simulink model "trackVehicleNewVer7_SonarPath"  (R2018b)
settings: Solver=ode45  StartTime=0.0  StopTime=100  FixedStep=0.1  RelTol=1e-3  EnableMultiTasking=on
PreLoadFcn:
  | RTWConfigurationCB('preloadfcn', bdroot);
InitFcn:
  | parameterVehicle
  | parameterObstacles
  | parameterGNC
  | parameterOccupancyGrid
  | parameterPathPlanner
  | parameterWaypointGenerator
  | miscParameters
StopFcn:
  | myAnimationSonarPath(xActEst,yActEst,thetaActEst,X_array, Y_array, rp1,rp2,sonarInfo, obstaclesArray, OccGrid, gridorig, cellsize)
values from neighbouring files (symbols this model uses):
  b = 0.32    [parameterVehicle.m]
  bDR = b    [parameterGNC.m]
  dcArray = [-uv -un-1 -un 0 un un+1 uv]    [parameterVehicle.m]
  dcArrayDR = [-uv -un-1 -un 0 un un+1 uv]    [parameterGNC.m]
  eTick = 1050    [parameterVehicle.m]
  eTickDR = eTick    [parameterGNC.m]
  KP1 = 8    [parameterGNC.m]
  KP2 = 20    [parameterGNC.m]
  maxgoaldist = 0.3    [parameterWaypointGenerator.m]
  maxwaydist = 0.5    [parameterWaypointGenerator.m]
  rl = 1*rNominal    (= 0.06)    [parameterVehicle.m]
  rNominal = 0.06    [parameterVehicle.m]
  rNominalDR = rNominal    [parameterGNC.m]
  rp1 = 0.3    [parameterGNC.m]
  rr = 1*rNominal    (= 0.06)    [parameterVehicle.m]
  Tau1 = 0.01    [parameterGNC.m]
  Tau2 = 0.1    [parameterGNC.m]
  TauEncoderDR = 0.1    [parameterGNC.m]
  thetaIC = 0*(pi/180)    (= 0)    [parameterVehicle.m]
  Tsample = 1/10    (= 0.1)    [parameterGNC.m]
  TsampleEncoder = 1/10    (= 0.1)    [parameterVehicle.m]
  TsampleEncoderDR = TsampleEncoder    [parameterGNC.m]
  Vcom = 1.5    [parameterGNC.m]
  wArray = [-Vmax, -Vmin, 0, 0,   0, Vmin, Vmax]./rNominal    [parameterVehicle.m]
  wArrayDR = [-Vmax, -Vmin, -Vmin/100, 0,   Vmin/100, Vmin, Vmax]./rNominal    [parameterGNC.m]
  xIC = 0    [parameterVehicle.m]
  yIC = 0    [parameterVehicle.m]
undefined symbols (not defined in the file or in its folder): DiscIntNeverNeededParam, obstaclesArray, sonar, X, Y, Z
libraries: robotlib x24, simulink x10, aerolibanimutils x1
CloseFcn:
  | rtwprivate ssgencode ModelCloseRequest track_vehicle6_v2
settings Model: Creator=Dogan  LastModifiedBy=uvs2
settings DataIOCC: LimitDataPoints=on  SaveFormat=Array  SignalLoggingSaveFormat=ModelDataLogs
settings OptimizationCC: ExpressionDepthLimit=2147483647  InitFltsAndDblsToZero=on  LifeSpan=inf
settings DebuggingCC: SaveWithParameterizedLinksMsg=none  UnderspecifiedInitializationDetection=Classic  MergeDetectMultiDrivingBlocksExec=none  SignalResolutionControl=TryResolveAllWithWarning  SolverPrmCheckMsg=warning  MultiTaskDSMMsg=warning  MultiTaskCondExecSysMsg=none  FcnCallInpInsideContextMsg=warning  StateNameClashWarn=warning  SFUnexpectedBacktrackingDiag=warning  SFNoUnconditionalDefaultTransitionDiag=warning  SFExecutionAtInitializationDiag=none
settings HardwareCC: ProdBitPerLong=64  ProdLargestAtomicFloat=None  ProdHWDeviceType=Intel->x86-64  TargetHWDeviceType=32-bit Generic
settings ModelReferenceCC: PropagateSignalLabelsOutOfModel=off
settings SFSimCC: SimUseLocalCustomCode=off  SimParseCustomCode=off
settings RTWCC: Description=Generic Real-Time Target  RTWUseLocalCustomCode=off
settings CodeAppCC: GenerateComments=off  SimulinkBlockComments=off
settings GRTTargetCC: TargetLangStandard=C89/C90 (ANSI)  GeneratePreprocessorConditionals=Disable all
settings ConfigComp: CovMetricSettings=dw  CovHtmlReporting=on  CovSaveCumulativeToWorkspaceVar=on  CovSaveSingleToWorkspaceVar=on  CovExternalEMLEnable=off

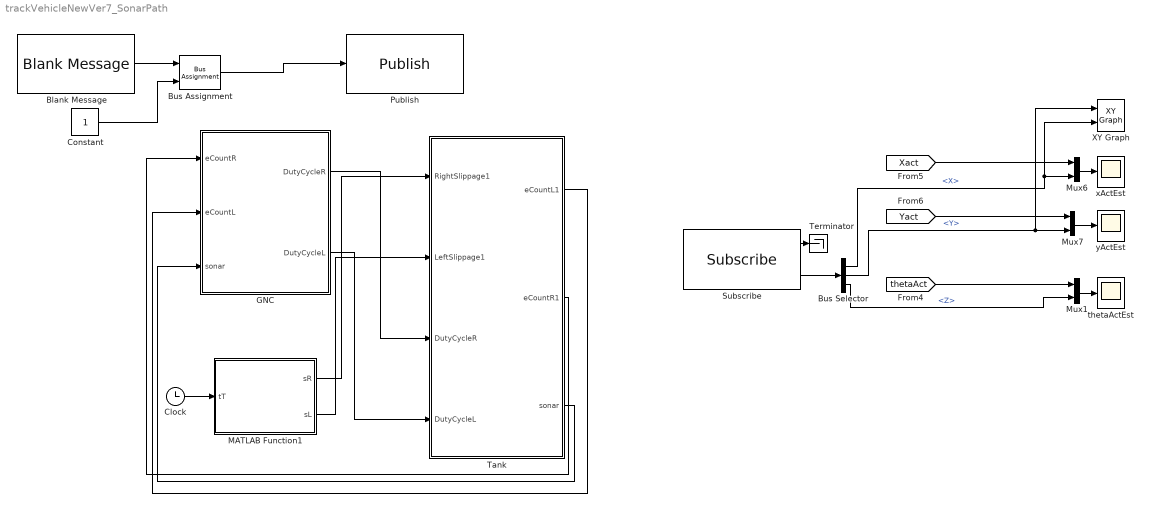
== system trackVehicleNewVer7_SonarPath ==
  Blank Message : robotlib/Blank Message  messageClass=Message  entityType=std_msgs/Bool  messageType=std_msgs/Bool  SampleTime=-1
      settings: SourceProductBaseCode=RO
  Bus Assignment : BusAssignment  AssignedSignals=Data
  Bus Selector : BusSelector  OutputSignals=X,Y,Z
  Clock : Clock
  Constant : Constant  OutDataTypeStr=boolean
  GNC : Subsystem
  MATLAB Function1 : MATLAB Function  TreatAsAtomicUnit=on
  Mux1 : Mux  Inputs=2
  Mux6 : Mux  Inputs=2
  Mux7 : Mux  Inputs=2
  Publish : robotlib/Publish  topicSource=Specify your own  topic=/start  messageType=std_msgs/Bool  messageQueueLength=1
      settings: SourceProductBaseCode=RO
  Subscribe : robotlib/Subscribe  topicSource=Specify your own  topic=/odometry  messageType=geometry_msgs/Point  sampleTime=-1  messageQueueLength=1
      settings: SourceProductBaseCode=RO
  Tank : Subsystem
  Terminator : Terminator
  XY Graph : simulink/Sinks/XY Graph  xmin=-1  xmax=9  ymin=-1  ymax=9  st=-1
  thetaActEst : Scope
  xActEst : Scope
  yActEst : Scope
  wires:
  Clock/1 -> MATLAB Function1/1(tT)
  Bus Selector/1 -> XY Graph/2, Mux6/2  "<X>"
  Mux6/1 -> xActEst/1
  Bus Selector/2 -> Mux7/2, XY Graph/1  "<Y>"
  [Xact] -> Mux6/1
  [Yact] -> Mux7/1
  Mux7/1 -> yActEst/1
  Bus Selector/3 -> Mux1/2  "<Z>"
  Mux1/1 -> thetaActEst/1
  [thetaAct] -> Mux1/1
  Subscribe/2 -> Bus Selector/1
  Blank Message/1 -> Bus Assignment/1
  Bus Assignment/1 -> Publish/1
  Constant/1 -> Bus Assignment/2
  Subscribe/1 -> Terminator/1
  GNC/1(DutyCycleR) -> Tank/3(DutyCycleR)
  GNC/2(DutyCycleL) -> Tank/4(DutyCycleL)
  MATLAB Function1/1(sR) -> Tank/1(RightSlippage1)
  MATLAB Function1/2(sL) -> Tank/2(LeftSlippage1)
  Tank/3(sonar) -> GNC/3(sonar)
  Tank/2("eCountR1 ") -> GNC/1(eCountR)
  Tank/1(eCountL1) -> GNC/2(eCountL)

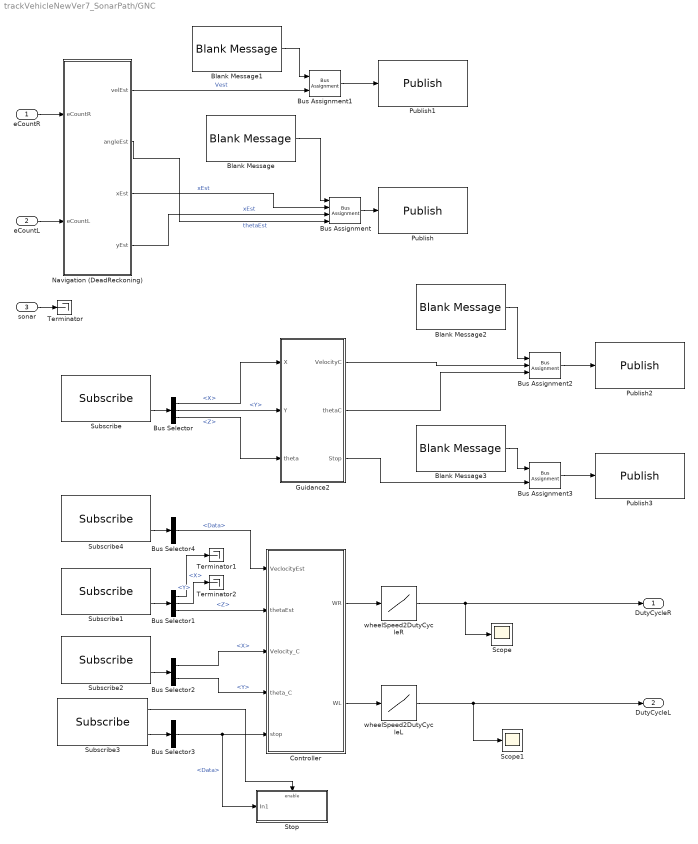
== system trackVehicleNewVer7_SonarPath/GNC ==
  eCountR : Inport
  eCountL : Inport  Port=2
  sonar : Inport  Port=3
  Blank Message : robotlib/Blank Message  messageClass=Message  entityType=geometry_msgs/Point  messageType=geometry_msgs/Point  SampleTime=inf
      settings: SourceProductBaseCode=RO
  Blank Message1 : robotlib/Blank Message  messageClass=Message  entityType=std_msgs/Float64  messageType=std_msgs/Float64  SampleTime=inf
      settings: SourceProductBaseCode=RO
  Blank Message2 : robotlib/Blank Message  messageClass=Message  entityType=geometry_msgs/Point  messageType=geometry_msgs/Point  SampleTime=inf
      settings: SourceProductBaseCode=RO
  Blank Message3 : robotlib/Blank Message  messageClass=Message  entityType=std_msgs/Bool  messageType=std_msgs/Bool  SampleTime=inf
      settings: SourceProductBaseCode=RO
  Bus Assignment : BusAssignment  AssignedSignals=X,Y,Z
  Bus Assignment1 : BusAssignment  AssignedSignals=Data
  Bus Assignment2 : BusAssignment  AssignedSignals=X,Y
  Bus Assignment3 : BusAssignment  AssignedSignals=Data
  Bus Selector : BusSelector  OutputSignals=X,Y,Z
  Bus Selector1 : BusSelector  OutputSignals=X,Y,Z
  Bus Selector2 : BusSelector  OutputSignals=X,Y
  Bus Selector3 : BusSelector  OutputSignals=Data
  Bus Selector4 : BusSelector  OutputSignals=Data
  Controller : Subsystem
  Guidance2 : Subsystem
  Navigation (DeadReckoning) : Subsystem
  Publish : robotlib/Publish  topicSource=Specify your own  topic=/odometry  messageType=geometry_msgs/Point  messageQueueLength=1
      settings: SourceProductBaseCode=RO
  Publish1 : robotlib/Publish  topicSource=Specify your own  topic=/velEst  messageType=std_msgs/Float64  messageQueueLength=1
      settings: SourceProductBaseCode=RO
  Publish2 : robotlib/Publish  topicSource=Specify your own  topic=/controlcommands  messageType=geometry_msgs/Point  messageQueueLength=1
      settings: SourceProductBaseCode=RO
  Publish3 : robotlib/Publish  topicSource=Specify your own  topic=/stop  messageType=std_msgs/Bool  messageQueueLength=1
      settings: SourceProductBaseCode=RO
  Scope : Scope
  Scope1 : Scope
  Stop : Subsystem  TreatAsAtomicUnit=on
  Subscribe : robotlib/Subscribe  topicSource=Specify your own  topic=/odometry  messageType=geometry_msgs/Point  sampleTime=-1  messageQueueLength=1
      settings: SourceProductBaseCode=RO
  Subscribe1 : robotlib/Subscribe  topicSource=Specify your own  topic=/odometry  messageType=geometry_msgs/Point  sampleTime=-1  messageQueueLength=1
      settings: SourceProductBaseCode=RO
  Subscribe2 : robotlib/Subscribe  topicSource=Specify your own  topic=/controlcommands  messageType=geometry_msgs/Point  sampleTime=-1  messageQueueLength=1
      settings: SourceProductBaseCode=RO
  Subscribe3 : robotlib/Subscribe  topicSource=Specify your own  topic=/stop  messageType=std_msgs/Bool  sampleTime=-1  messageQueueLength=1
      settings: SourceProductBaseCode=RO
  Subscribe4 : robotlib/Subscribe  topicSource=Specify your own  topic=/velEst  messageType=std_msgs/Float64  sampleTime=-1  messageQueueLength=1
      settings: SourceProductBaseCode=RO
  Terminator : Terminator
  Terminator1 : Terminator
  Terminator2 : Terminator
  wheelSpeed2DutyCycleL : Lookup  InputValues=wArrayDR  Table=dcArrayDR  LookUpMeth=Interpolation-Use End Values
  wheelSpeed2DutyCycleR : Lookup  InputValues=wArrayDR  Table=dcArrayDR  LookUpMeth=Interpolation-Use End Values
  DutyCycleR : Outport
  DutyCycleL : Outport  Port=2
  wires:
  Controller/2(WL) -> wheelSpeed2DutyCycleL/1
  Guidance2/2(thetaC) -> Bus Assignment2/3
  Guidance2/1(VelocityC) -> Bus Assignment2/2
  eCountR/1 -> Navigation (DeadReckoning)/1(eCountR)
  eCountL/1 -> Navigation (DeadReckoning)/2(eCountL)
  Navigation (DeadReckoning)/1(velEst) -> Bus Assignment1/2  "Vest"
  Navigation (DeadReckoning)/2(angleEst) -> Bus Assignment/4  "thetaEst"
  Navigation (DeadReckoning)/3(xEst) -> Bus Assignment/2  "xEst"
  Navigation (DeadReckoning)/4(yEst) -> Bus Assignment/3  "xEst"
  Controller/1(WR) -> wheelSpeed2DutyCycleR/1
  Guidance2/3(Stop) -> Bus Assignment3/2
  sonar/1 -> Terminator/1
  Bus Assignment/1 -> Publish/1
  Blank Message/1 -> Bus Assignment/1
  Blank Message1/1 -> Bus Assignment1/1
  Bus Assignment1/1 -> Publish1/1
  Subscribe/2 -> Bus Selector/1
  Bus Selector/1 -> Guidance2/1(X)  "<X>"
  Bus Selector/2 -> Guidance2/2(Y)  "<Y>"
  Bus Selector/3 -> Guidance2/3(theta)  "<Z>"
  Bus Assignment2/1 -> Publish2/1
  Blank Message2/1 -> Bus Assignment2/1
  Subscribe1/2 -> Bus Selector1/1
  Bus Selector1/3 -> Controller/2(thetaEst)  "<Z>"
  Bus Selector1/1 -> Terminator1/1  "<X>"
  Bus Selector1/2 -> Terminator2/1  "<Y>"
  Subscribe2/2 -> Bus Selector2/1
  Bus Selector2/1 -> Controller/3(Velocity_C)  "<X>"
  Bus Selector2/2 -> Controller/4(theta_C)  "<Y>"
  Bus Assignment3/1 -> Publish3/1
  Blank Message3/1 -> Bus Assignment3/1
  Subscribe3/2 -> Bus Selector3/1
  Bus Selector3/1 -> Stop/1(In1), Controller/5(stop)  "<Data>"
  Subscribe4/2 -> Bus Selector4/1
  Bus Selector4/1 -> Controller/1(VeclocityEst)  "<Data>"
  Subscribe3/1 -> Stop/Enable
  wheelSpeed2DutyCycleR/1 -> Scope/1, DutyCycleR/1
  wheelSpeed2DutyCycleL/1 -> Scope1/1, DutyCycleL/1

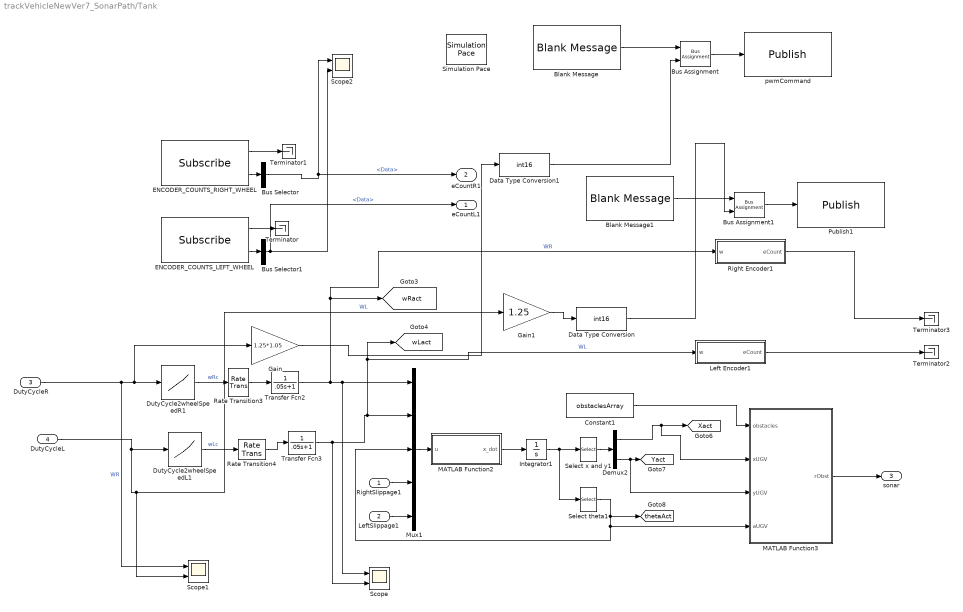
== system trackVehicleNewVer7_SonarPath/Tank ==
  RightSlippage1 : Inport
  LeftSlippage1 : Inport  Port=2
  DutyCycleR : Inport  Port=3
  DutyCycleL : Inport  Port=4
  Blank Message : robotlib/Blank Message  messageClass=Message  entityType=std_msgs/Int16  messageType=std_msgs/Int16  SampleTime=inf
      settings: SourceProductBaseCode=RO
  Blank Message1 : robotlib/Blank Message  messageClass=Message  entityType=std_msgs/Int16  messageType=std_msgs/Int16  SampleTime=inf
      settings: SourceProductBaseCode=RO
  Bus Assignment : BusAssignment  AssignedSignals=Data
  Bus Assignment1 : BusAssignment  AssignedSignals=Data
  Bus Selector : BusSelector  OutputSignals=Data
  Bus Selector1 : BusSelector  OutputSignals=Data
  Constant1 : Constant  Value=obstaclesArray
  Data Type Conversion : DataTypeConversion  OutDataTypeStr=int16
  Data Type Conversion1 : DataTypeConversion  OutDataTypeStr=int16
  Demux2 : Demux  Outputs=2
  DutyCycle2wheelSpeedL1 : Lookup  InputValues=dcArray  Table=wArray  LookUpMeth=Interpolation-Use End Values
  DutyCycle2wheelSpeedR1 : Lookup  InputValues=dcArray  Table=wArray  LookUpMeth=Interpolation-Use End Values
  ENCODER_COUNTS_LEFT_WHEEL : robotlib/Subscribe  topicSource=Select from ROS network  topic=/enco_L  messageType=std_msgs/Int16  sampleTime=-1  messageQueueLength=1
      settings: SourceProductBaseCode=RO
  ENCODER_COUNTS_RIGHT_WHEEL : robotlib/Subscribe  topicSource=Select from ROS network  topic=/enco_R  messageType=std_msgs/Int16  sampleTime=-1  messageQueueLength=1
      settings: SourceProductBaseCode=RO
  Gain : Gain  Gain=1.25*1.05
  Gain1 : Gain  Gain=1.25
  Integrator1 : Integrator  InitialCondition=[xIC; yIC ; thetaIC]
  Left Encoder1 : Subsystem
  MATLAB Function2 : MATLAB Function  TreatAsAtomicUnit=on
  MATLAB Function3 : MATLAB Function  TreatAsAtomicUnit=on  SystemSampleTime=sonar.Ts
  Mux1 : Mux  Inputs=5
  Publish1 : robotlib/Publish  topicSource=Select from ROS network  topic=/pwm_cmd_l  messageType=std_msgs/Int16  messageQueueLength=1
      settings: SourceProductBaseCode=RO
  Rate Transition3 : RateTransition
  Rate Transition4 : RateTransition  OutPortSampleTimeOpt=Inherit
  Right Encoder1 : Subsystem
  Scope : Scope  NumInputPorts=2
  Scope1 : Scope  NumInputPorts=2
  Scope2 : Scope  NumInputPorts=2
  Select theta1 : Selector  InputPortWidth=3  IndexOptions=Index vector (dialog)  Indices=3  OutputSizes=1
  Select x and y1 : Selector  InputPortWidth=3  IndexOptions=Index vector (dialog)  Indices=[1 2]  OutputSizes=1
  Simulation Pace : aerolibanimutils/Simulation Pace  SimulationPace=1  SleepMode=MATLAB Thread  OutputPaceError=off  SampleTime=1/30
  Terminator{,1..3} (4 alike) : Terminator
  Transfer Fcn2 : TransferFcn  Denominator=[.05 1]
  Transfer Fcn3 : TransferFcn  Denominator=[.05 1]
  pwmCommand : robotlib/Publish  topicSource=Select from ROS network  topic=/pwm_cmd_r  messageType=std_msgs/Int16  messageQueueLength=1
      settings: SourceProductBaseCode=RO
  eCountL1 : Outport
  "eCountR1 " : Outport  Port=2
  sonar : Outport  Port=3
  tag scope: Xact=global, Yact=global, thetaAct=global, wLact=global, wRact=global
  wires:
  Select theta1/1 -> MATLAB Function3/4(aUGV), Mux1/3, [thetaAct]
  Demux2/1 -> MATLAB Function3/2(xUGV), [Xact]
  Data Type Conversion1/1 -> Bus Assignment/2
  Data Type Conversion/1 -> Bus Assignment1/2
  DutyCycleL/1 -> DutyCycle2wheelSpeedL1/1, Scope1/2, Gain1/1  "WL"
  RightSlippage1/1 -> Mux1/4
  Left Encoder1/1(eCount) -> Terminator2/1
  Rate Transition4/1 -> Transfer Fcn3/1
  Mux1/1 -> MATLAB Function2/1(u)
  Gain1/1 -> Data Type Conversion/1
  Blank Message/1 -> Bus Assignment/1
  ENCODER_COUNTS_LEFT_WHEEL/2 -> Bus Selector1/1
  Demux2/2 -> MATLAB Function3/3(yUGV), [Yact]
  LeftSlippage1/1 -> Mux1/5
  DutyCycle2wheelSpeedL1/1 -> Rate Transition4/1  "wLc"
  Transfer Fcn3/1 -> Scope/2, Left Encoder1/1(w), [wLact], Mux1/2  "WL"
  ENCODER_COUNTS_RIGHT_WHEEL/2 -> Bus Selector/1
  Gain/1 -> Data Type Conversion1/1
  Bus Assignment1/1 -> Publish1/1
  Blank Message1/1 -> Bus Assignment1/1
  ENCODER_COUNTS_RIGHT_WHEEL/1 -> Terminator1/1
  Bus Assignment/1 -> pwmCommand/1
  Transfer Fcn2/1 -> [wRact], Right Encoder1/1(w), Scope/1, Mux1/1  "WR"
  Rate Transition3/1 -> Transfer Fcn2/1
  Integrator1/1 -> Select theta1/1, Select x and y1/1
  Bus Selector1/1 -> Scope2/2, eCountL1/1  "<Data>"
  MATLAB Function2/1(x_dot) -> Integrator1/1
  DutyCycleR/1 -> Scope1/1, Gain/1, DutyCycle2wheelSpeedR1/1  "WR"
  Bus Selector/1 -> "eCountR1 "/1, Scope2/1  "<Data>"
  ENCODER_COUNTS_LEFT_WHEEL/1 -> Terminator/1
  Right Encoder1/1(eCount) -> Terminator3/1
  DutyCycle2wheelSpeedR1/1 -> Rate Transition3/1  "wRc"
  Select x and y1/1 -> Demux2/1
  Constant1/1 -> MATLAB Function3/1(obstacles)
  MATLAB Function3/1(rObst) -> sonar/1

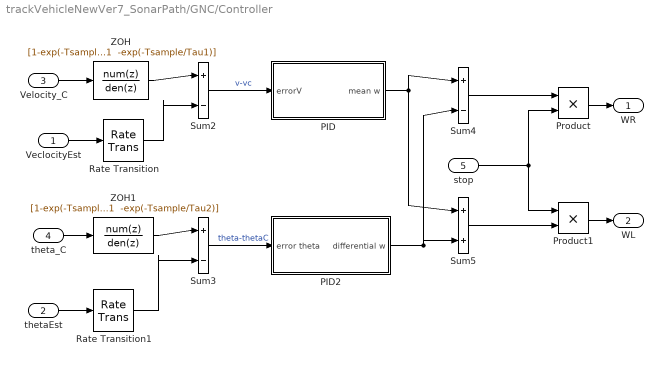
== system trackVehicleNewVer7_SonarPath/GNC/Controller ==
  VeclocityEst : Inport
  thetaEst : Inport  Port=2
  Velocity_C : Inport  Port=3
  theta_C : Inport  Port=4
  stop : Inport  Port=5
  PID : Subsystem
  PID2 : Subsystem
  Product : Product  RndMeth=Zero
  Product1 : Product  RndMeth=Zero
  Rate Transition : RateTransition  Deterministic=off
  Rate Transition1 : RateTransition  Deterministic=off
  Sum2 : Sum  Inputs=|+|-|  SampleTime=Tsample
  Sum3 : Sum  Inputs=|+|-|  SampleTime=Tsample
  Sum4 : Sum  Inputs=+|-
  Sum5 : Sum  Inputs=+|+
  ZOH : DiscreteTransferFcn  Numerator=[1-exp(-Tsample/Tau1)]  Denominator="[1  -exp(-Tsample/Tau1)]"  SampleTime=Tsample
  ZOH1 : DiscreteTransferFcn  Numerator=[1-exp(-Tsample/Tau2)]  Denominator="[1  -exp(-Tsample/Tau2)]"  SampleTime=Tsample
  WR : Outport
  WL : Outport  Port=2
  wires:
  Rate Transition1/1 -> Sum3/2
  ZOH1/1 -> Sum3/1
  Rate Transition/1 -> Sum2/2
  ZOH/1 -> Sum2/1
  Sum3/1 -> PID2/1(error theta)  "theta-thetaC"
  Sum2/1 -> PID/1(errorV)  "v-vc"
  VeclocityEst/1 -> Rate Transition/1
  Velocity_C/1 -> ZOH/1
  thetaEst/1 -> Rate Transition1/1
  theta_C/1 -> ZOH1/1
  PID/1(mean w) -> Sum4/1, Sum5/1
  PID2/1(differential w) -> Sum4/2, Sum5/2
  Sum4/1 -> Product/1
  stop/1 -> Product1/1, Product/2
  Sum5/1 -> Product1/2
  Product/1 -> WR/1
  Product1/1 -> WL/1

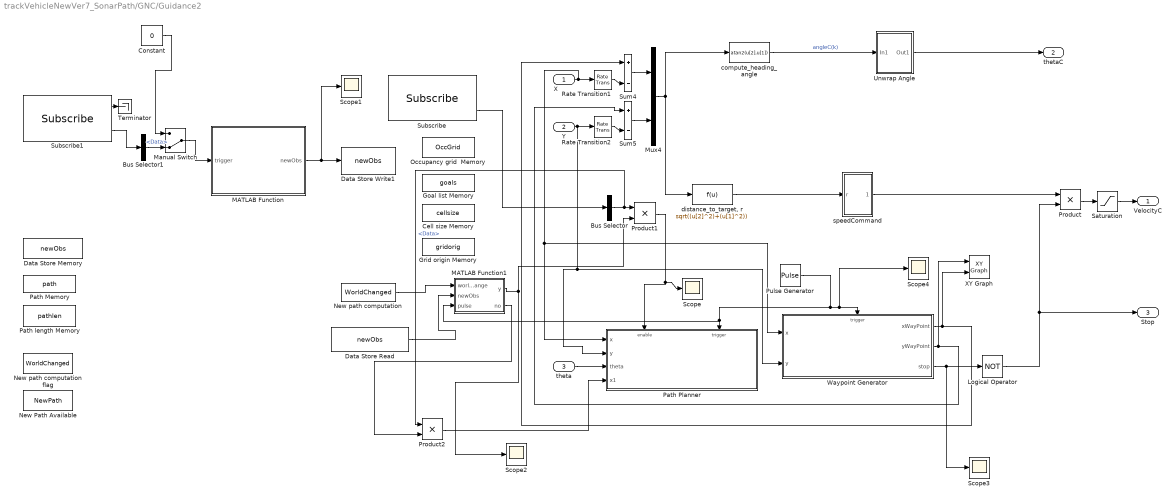
== system trackVehicleNewVer7_SonarPath/GNC/Guidance2 ==
  X : Inport
  Y : Inport  Port=2
  theta : Inport  Port=3
  Bus Selector : BusSelector  OutputSignals=Data
  Bus Selector1 : BusSelector  OutputSignals=Data
  Cell size Memory : DataStoreMemory  DataStoreName=cellsize  ReadBeforeWriteMsg=warning  WriteAfterWriteMsg=warning  WriteAfterReadMsg=warning  InitialValue=cellsize  VectorParams1D=off  ShowAdditionalParam=off
  Constant : Constant  Value=0
  Data Store Memory : DataStoreMemory  DataStoreName=newObs  ReadBeforeWriteMsg=warning  WriteAfterWriteMsg=warning  WriteAfterReadMsg=warning  ShowAdditionalParam=off
  Data Store Read : DataStoreRead  DataStoreName=newObs
  Data Store Write1 : DataStoreWrite  DataStoreName=newObs
  Goal list Memory : DataStoreMemory  DataStoreName=goals  ReadBeforeWriteMsg=warning  WriteAfterWriteMsg=warning  WriteAfterReadMsg=warning  InitialValue=goals  VectorParams1D=off  ShowAdditionalParam=off
  Grid origin Memory : DataStoreMemory  DataStoreName=gridorig  InitialValue=gridorig  VectorParams1D=off  ShowAdditionalParam=off
  Logical Operator : Logic  Operator=NOT  AllPortsSameDT=off
  MATLAB Function : MATLAB Function  TreatAsAtomicUnit=on
  MATLAB Function1 : MATLAB Function  TreatAsAtomicUnit=on
  Manual Switch : ManualSwitch  CurrentSetting=0
  Mux4 : Mux  Inputs=2
  New Path Available : DataStoreMemory  DataStoreName=NewPath  ReadBeforeWriteMsg=warning  WriteAfterWriteMsg=warning  WriteAfterReadMsg=warning  VectorParams1D=off  ShowAdditionalParam=off
  New path computation : DataStoreRead  DataStoreName=WorldChanged
  New path computation flag : DataStoreMemory  DataStoreName=WorldChanged  InitialValue=WorldChanged  VectorParams1D=off  ShowAdditionalParam=off
  Occupancy grid  Memory : DataStoreMemory  DataStoreName=OccGrid  InitialValue=OccGrid  VectorParams1D=off  ShowAdditionalParam=off
  Path Memory : DataStoreMemory  DataStoreName=path  InitialValue=path  VectorParams1D=off  ShowAdditionalParam=off
  Path Planner : Subsystem
  Path length Memory : DataStoreMemory  DataStoreName=pathlen  InitialValue=pathlen  VectorParams1D=off  ShowAdditionalParam=off
  Product : Product  RndMeth=Zero
  Product1 : Product
  Product2 : Product
  Pulse Generator : DiscretePulseGenerator  PulseType=Time based  Period=0.1  PulseWidth=5
  Rate Transition1 : RateTransition
  Rate Transition2 : RateTransition
  Saturation : Saturate  UpperLimit=Vcom  LowerLimit=0  SampleTime=Tsample
  Scope{,1..4} (5 alike) : Scope
  Subscribe : robotlib/Subscribe  topicSource=Specify your own  topic=/start  messageType=std_msgs/Bool  sampleTime=-1  messageQueueLength=1
      settings: SourceProductBaseCode=RO
  Subscribe1 : robotlib/Subscribe  topicSource=Select from ROS network  topic=/axisX  messageType=std_msgs/Int32  sampleTime=-1  messageQueueLength=1
      settings: SourceProductBaseCode=RO
  Sum4 : Sum  Inputs=|+|-|
  Sum5 : Sum  Inputs=|+|-|
  Terminator : Terminator
  Unwrap Angle : Subsystem
  Waypoint Generator : Subsystem
  XY Graph : simulink/Sinks/XY Graph  xmin=-1  xmax=9  ymin=-1  ymax=9  st=-1
  compute_heading_angle : Fcn  Expr=atan2(u[2],u[1])  SampleTime=Tsample
  "distance_to_target, r" : Fcn  Expr=sqrt((u[2]^2)+(u[1]^2))  SampleTime=Tsample
  speedCommand : Subsystem
  VelocityC : Outport
  thetaC : Outport  Port=2
  Stop : Outport  Port=3
  wires:
  Product/1 -> Saturation/1
  Rate Transition2/1 -> Sum5/2
  Rate Transition1/1 -> Sum4/2
  Unwrap Angle/1(Out1) -> thetaC/1
  Saturation/1 -> VelocityC/1
  Sum5/1 -> Mux4/2
  Y/1 -> Rate Transition2/1, Path Planner/2(y), Waypoint Generator/2(y)
  X/1 -> Rate Transition1/1, Waypoint Generator/1(x), Path Planner/1(x)
  Mux4/1 -> "distance_to_target, r"/1, compute_heading_angle/1
  "distance_to_target, r"/1 -> speedCommand/1(r)
  Sum4/1 -> Mux4/1
  compute_heading_angle/1 -> Unwrap Angle/1(In1)  "angleC(k)"
  speedCommand/1(Vdes) -> Product/1
  theta/1 -> Path Planner/3(theta)
  Waypoint Generator/1(xWayPoint) -> XY Graph/2, Sum4/1
  Waypoint Generator/2(yWayPoint) -> XY Graph/1, Sum5/1
  Waypoint Generator/3(stop) -> Scope3/1, Logical Operator/1
  Logical Operator/1 -> Stop/1, Product/2
  Product1/1 -> Scope/1, Path Planner/Enable
  Subscribe/2 -> Bus Selector/1
  MATLAB Function/1(newObs) -> Scope1/1, Data Store Write1/1
  Data Store Read/1 -> MATLAB Function1/2(newObs)
  MATLAB Function1/1(y) -> Scope2/1, Product1/2
  New path computation/1 -> MATLAB Function1/1(worldChange)
  Pulse Generator/1 -> MATLAB Function1/3(pulse), Path Planner/Trigger, Scope4/1, Waypoint Generator/Trigger
  Bus Selector/1 -> Product2/1, Product1/1  "<Data>"
  MATLAB Function1/2(no) -> Product2/2
  Product2/1 -> Path Planner/4(x1)
  Subscribe1/2 -> Bus Selector1/1
  Subscribe1/1 -> Terminator/1
  Bus Selector1/1 -> Manual Switch/2  "<Data>"
  Manual Switch/1 -> MATLAB Function/1(trigger)
  Constant/1 -> Manual Switch/1

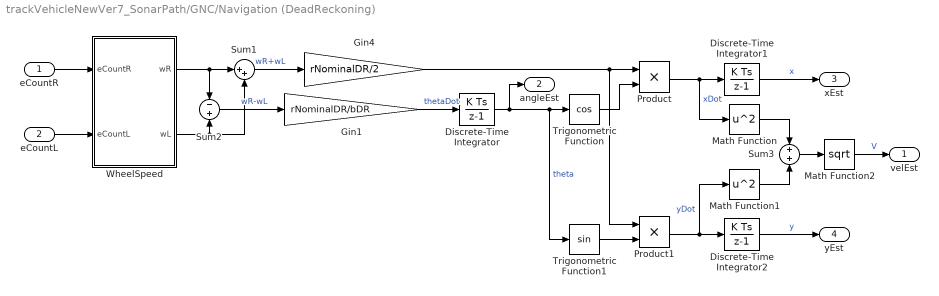
== system trackVehicleNewVer7_SonarPath/GNC/Navigation (DeadReckoning) ==
  eCountR : Inport
  eCountL : Inport  Port=2
  Discrete-Time Integrator : DiscreteIntegrator  SampleTime=TsampleEncoderDR  ICPrevOutput=DiscIntNeverNeededParam  ICPrevScaledInput=DiscIntNeverNeededParam
  Discrete-Time Integrator1 : DiscreteIntegrator  SampleTime=TsampleEncoderDR  ICPrevOutput=DiscIntNeverNeededParam  ICPrevScaledInput=DiscIntNeverNeededParam
  Discrete-Time Integrator2 : DiscreteIntegrator  SampleTime=TsampleEncoderDR  ICPrevOutput=DiscIntNeverNeededParam  ICPrevScaledInput=DiscIntNeverNeededParam
  Gin1 : Gain  Gain=rNominalDR/bDR  OutDataTypeStr=double
  Gin4 : Gain  Gain=rNominalDR/2  OutDataTypeStr=double
  Math Function : Math  Operator=square  SaturateOnIntegerOverflow=on
  Math Function1 : Math  Operator=square  SaturateOnIntegerOverflow=on
  Math Function2 : Math  Operator=sqrt  OutputSignalType=real  SaturateOnIntegerOverflow=on
  Product : Product  RndMeth=Zero
  Product1 : Product  RndMeth=Zero
  Sum1 : Sum  Inputs=|++
  Sum2 : Sum  Inputs=-|+
  Sum3 : Sum  Inputs=+|+
  Trigonometric Function : Trigonometry  Operator=cos  OutputSignalType=real
  Trigonometric Function1 : Trigonometry  OutputSignalType=real
  WheelSpeed : Subsystem
  velEst : Outport
  angleEst : Outport  Port=2
  xEst : Outport  Port=3
  yEst : Outport  Port=4
  wires:
  eCountR/1 -> WheelSpeed/1(eCountR)
  eCountL/1 -> WheelSpeed/2(eCountL)
  WheelSpeed/2(wL) -> Sum1/2, Sum2/2
  WheelSpeed/1(wR) -> Sum1/1, Sum2/1
  Sum1/1 -> Gin4/1  "wR+wL"
  Sum2/1 -> Gin1/1  "wR-wL"
  Gin1/1 -> Discrete-Time Integrator/1  "thetaDot"
  Discrete-Time Integrator/1 -> Trigonometric Function/1, Trigonometric Function1/1, angleEst/1  "theta"
  Trigonometric Function/1 -> Product/2
  Gin4/1 -> Product/1, Product1/1
  Trigonometric Function1/1 -> Product1/2
  Product/1 -> Discrete-Time Integrator1/1, Math Function/1  "xDot"
  Product1/1 -> Discrete-Time Integrator2/1, Math Function1/1  "yDot"
  Discrete-Time Integrator1/1 -> xEst/1  "x"
  Discrete-Time Integrator2/1 -> yEst/1  "y"
  Math Function/1 -> Sum3/1
  Math Function1/1 -> Sum3/2
  Sum3/1 -> Math Function2/1
  Math Function2/1 -> velEst/1  "V"

== system trackVehicleNewVer7_SonarPath/GNC/Stop ==
  In1 : Inport
  Enable : EnablePort
  Compare To Zero : simulink/Logic and Bit Operations/Compare To Zero  relop===  OutDataTypeStr=boolean
  Stop Simulation : Stop
  wires:
  Compare To Zero/1 -> Stop Simulation/1
  In1/1 -> Compare To Zero/1

== system trackVehicleNewVer7_SonarPath/Tank/Left Encoder1 ==
  w : Inport
  Rate Transition1 : RateTransition
  WheelAngleL : Integrator
  angle2tick2 : Gain  Gain=eTick*rNominal  OutDataTypeStr=int16  SampleTime=TsampleEncoder
  eCount : Outport
  wires:
  WheelAngleL/1 -> Rate Transition1/1  "gammaL"
  w/1 -> WheelAngleL/1
  angle2tick2/1 -> eCount/1  "eCountL"
  Rate Transition1/1 -> angle2tick2/1

== system trackVehicleNewVer7_SonarPath/Tank/Right Encoder1 ==
  w : Inport
  Rate Transition1 : RateTransition
  WheelAngleR : Integrator
  angle2tick1 : Gain  Gain=eTick*rNominal  OutDataTypeStr=int16  SampleTime=TsampleEncoder
  eCount : Outport
  wires:
  WheelAngleR/1 -> Rate Transition1/1  "gammaR"
  w/1 -> WheelAngleR/1
  angle2tick1/1 -> eCount/1  "eCountR"
  Rate Transition1/1 -> angle2tick1/1

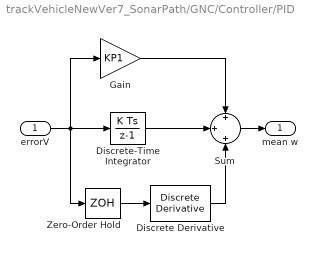
== system trackVehicleNewVer7_SonarPath/GNC/Controller/PID ==
  errorV : Inport
  Discrete Derivative : simulink/Discrete/Discrete Derivative  gainval=KD1  ICPrevScaledInput=0.0  OutMin=[]  OutMax=[]  OutDataType=sfix(16)  OutScaling=2^-10  DoSatur=off
  Discrete-Time Integrator : DiscreteIntegrator  gainval=KI1  SampleTime=Tsample  ICPrevOutput=DiscIntNeverNeededParam  ICPrevScaledInput=DiscIntNeverNeededParam
  Gain : Gain  Gain=KP1  SampleTime=Tsample
  Sum : Sum  Inputs=+|+|+
  Zero-Order Hold : ZeroOrderHold  SampleTime=Tsample
  mean w : Outport
  wires:
  Sum/1 -> mean w/1
  errorV/1 -> Zero-Order Hold/1, Gain/1, Discrete-Time Integrator/1
  Gain/1 -> Sum/1
  Discrete-Time Integrator/1 -> Sum/2
  Zero-Order Hold/1 -> Discrete Derivative/1
  Discrete Derivative/1 -> Sum/3

== system trackVehicleNewVer7_SonarPath/GNC/Controller/PID2 ==
  error theta : Inport
  Discrete Derivative1 : simulink/Discrete/Discrete Derivative  gainval=KD2  ICPrevScaledInput=0.0  OutMin=[]  OutMax=[]  OutDataType=sfix(16)  OutScaling=2^-10  DoSatur=off
  Discrete-Time Integrator1 : DiscreteIntegrator  gainval=KI2  SampleTime=Tsample  ICPrevOutput=DiscIntNeverNeededParam  ICPrevScaledInput=DiscIntNeverNeededParam
  Gain1 : Gain  Gain=KP2  SampleTime=Tsample
  Sum1 : Sum  Inputs=+|+|+
  Zero-Order Hold1 : ZeroOrderHold  SampleTime=Tsample
  differential w : Outport
  wires:
  Sum1/1 -> differential w/1
  Gain1/1 -> Sum1/1
  Discrete-Time Integrator1/1 -> Sum1/2
  error theta/1 -> Zero-Order Hold1/1, Discrete-Time Integrator1/1, Gain1/1
  Zero-Order Hold1/1 -> Discrete Derivative1/1
  Discrete Derivative1/1 -> Sum1/3

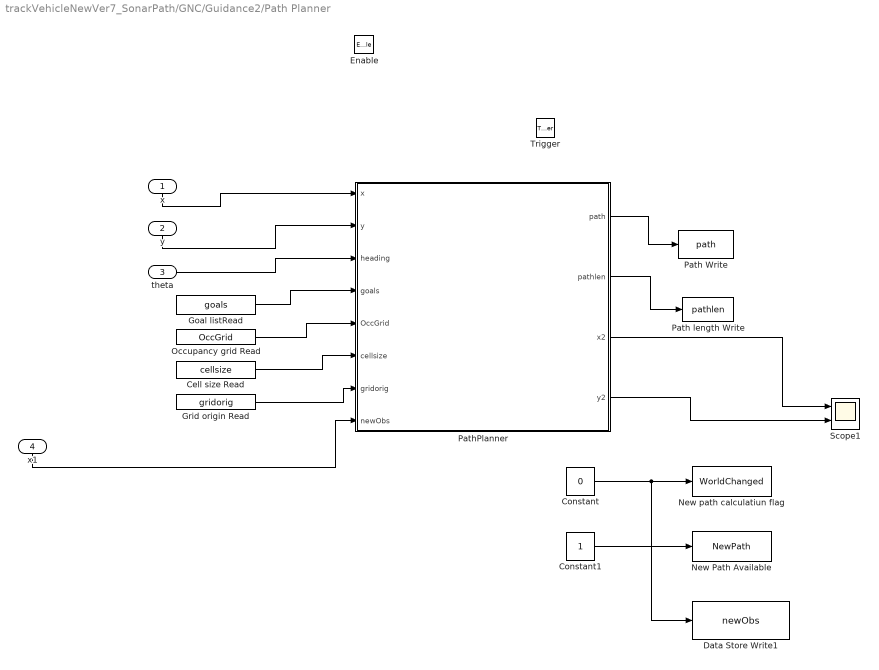
== system trackVehicleNewVer7_SonarPath/GNC/Guidance2/Path Planner ==
  x : Inport
  y : Inport  Port=2
  theta : Inport  Port=3
  x1 : Inport  Port=4
  Enable : EnablePort  ZeroCross=off
  Trigger : TriggerPort  VariantControl=(inherit)  PortDimensions=1
  Cell size Read : DataStoreRead  DataStoreName=cellsize
  Constant : Constant  Value=0  VectorParams1D=off
  Constant1 : Constant
  Data Store Write1 : DataStoreWrite  DataStoreName=newObs
  Goal listRead : DataStoreRead  DataStoreName=goals
  Grid origin Read : DataStoreRead  DataStoreName=gridorig
  New Path Available : DataStoreWrite  DataStoreName=NewPath
  New path calculatiun flag : DataStoreWrite  DataStoreName=WorldChanged  DataStoreElements=WorldChanged
  Occupancy grid Read : DataStoreRead  DataStoreName=OccGrid
  Path Write : DataStoreWrite  DataStoreName=path
  Path length Write : DataStoreWrite  DataStoreName=pathlen
  PathPlanner : MATLAB Function  TreatAsAtomicUnit=on
  Scope1 : Scope  NumInputPorts=2
  wires:
  theta/1 -> PathPlanner/3(heading)
  Grid origin Read/1 -> PathPlanner/7(gridorig)
  Cell size Read/1 -> PathPlanner/6(cellsize)
  Occupancy grid Read/1 -> PathPlanner/5(OccGrid)
  Goal listRead/1 -> PathPlanner/4(goals)
  x/1 -> PathPlanner/1(x)
  PathPlanner/1(path) -> Path Write/1
  Constant/1 -> Data Store Write1/1, New path calculatiun flag/1
  PathPlanner/2(pathlen) -> Path length Write/1
  Constant1/1 -> New Path Available/1
  y/1 -> PathPlanner/2(y)
  x1/1 -> PathPlanner/8(newObs)
  PathPlanner/4(y2) -> Scope1/2
  PathPlanner/3(x2) -> Scope1/1

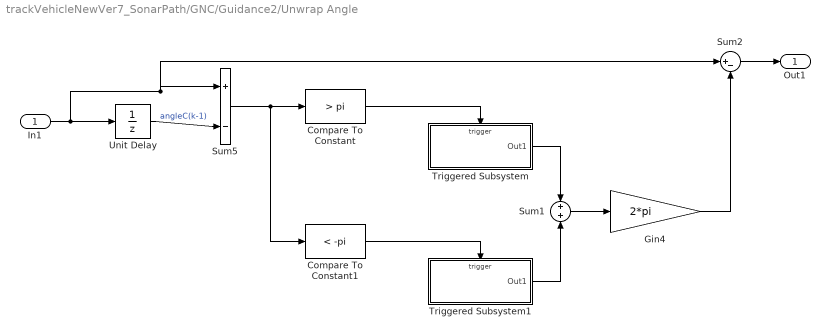
== system trackVehicleNewVer7_SonarPath/GNC/Guidance2/Unwrap Angle ==
  In1 : Inport
  Compare To Constant : simulink/Logic and Bit Operations/Compare To Constant  relop=>  const=pi  OutDataTypeStr=uint8  ZeroCross=off
  Compare To Constant1 : simulink/Logic and Bit Operations/Compare To Constant  relop=<  const=-pi  OutDataTypeStr=uint8  ZeroCross=off
  Gin4 : Gain  Gain=2*pi  OutDataTypeStr=double  SampleTime=Tsample
  Sum1 : Sum  Inputs=+|+
  Sum2 : Sum  Inputs=|+-
  Sum5 : Sum  Inputs=|+|-|
  Triggered Subsystem : Subsystem  TreatAsAtomicUnit=on
  Triggered Subsystem1 : Subsystem  TreatAsAtomicUnit=on
  Unit Delay : UnitDelay  SampleTime=Tsample
  Out1 : Outport
  wires:
  Gin4/1 -> Sum2/2
  Sum2/1 -> Out1/1
  Sum1/1 -> Gin4/1
  Triggered Subsystem1/1(Out1) -> Sum1/2
  Triggered Subsystem/1(Out1) -> Sum1/1
  Compare To Constant/1 -> Triggered Subsystem/Trigger
  Compare To Constant1/1 -> Triggered Subsystem1/Trigger
  Sum5/1 -> Compare To Constant1/1, Compare To Constant/1
  Unit Delay/1 -> Sum5/2  "angleC(k-1)"
  In1/1 -> Sum2/1, Sum5/1, Unit Delay/1

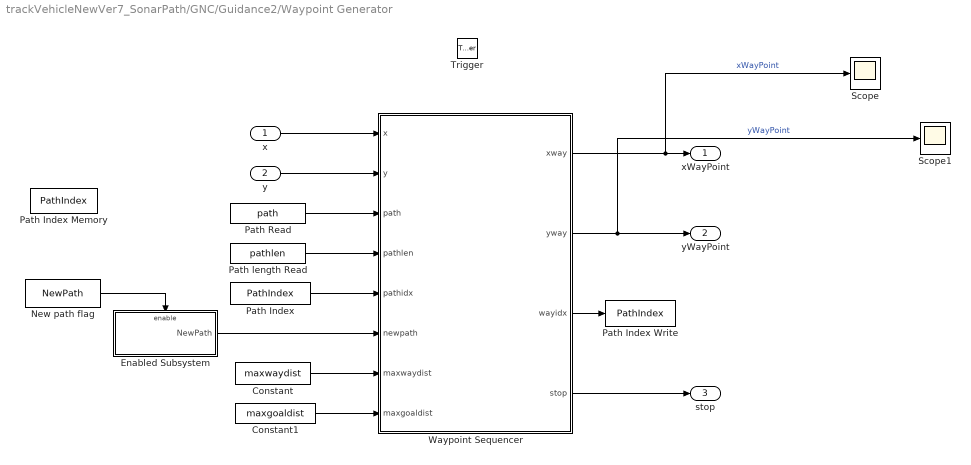
== system trackVehicleNewVer7_SonarPath/GNC/Guidance2/Waypoint Generator ==
  x : Inport
  y : Inport  Port=2
  Trigger : TriggerPort  VariantControl=(inherit)  PortDimensions=1
  Constant : Constant  Value=maxwaydist  VectorParams1D=off
  Constant1 : Constant  Value=maxgoaldist
  Enabled Subsystem : Subsystem  TreatAsAtomicUnit=on
  New path flag : DataStoreRead  DataStoreName=NewPath
  Path Index : DataStoreRead  DataStoreName=PathIndex
  Path Index Memory : DataStoreMemory  DataStoreName=PathIndex  InitialValue=1  VectorParams1D=off  ShowAdditionalParam=off
  Path Index Write : DataStoreWrite  DataStoreName=PathIndex
  Path Read : DataStoreRead  DataStoreName=path
  Path length Read : DataStoreRead  DataStoreName=pathlen
  Scope : Scope
  Scope1 : Scope
  Waypoint Sequencer : MATLAB Function  TreatAsAtomicUnit=on
  xWayPoint : Outport
  yWayPoint : Outport  Port=2
  stop : Outport  Port=3
  wires:
  Waypoint Sequencer/2(yway) -> Scope1/1, yWayPoint/1  "yWayPoint"
  Waypoint Sequencer/1(xway) -> Scope/1, xWayPoint/1  "xWayPoint"
  Path Read/1 -> Waypoint Sequencer/3(path)
  Path length Read/1 -> Waypoint Sequencer/4(pathlen)
  Path Index/1 -> Waypoint Sequencer/5(pathidx)
  Waypoint Sequencer/3(wayidx) -> Path Index Write/1
  New path flag/1 -> Enabled Subsystem/Enable
  Enabled Subsystem/1(NewPath) -> Waypoint Sequencer/6(newpath)
  Waypoint Sequencer/4(stop) -> stop/1
  Constant/1 -> Waypoint Sequencer/7(maxwaydist)
  Constant1/1 -> Waypoint Sequencer/8(maxgoaldist)
  y/1 -> Waypoint Sequencer/2(y)
  x/1 -> Waypoint Sequencer/1(x)

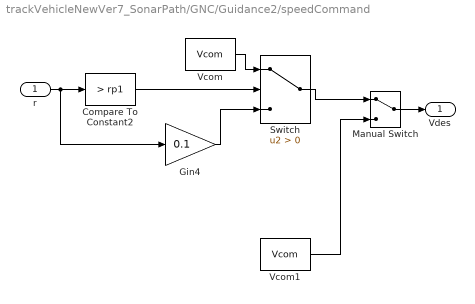
== system trackVehicleNewVer7_SonarPath/GNC/Guidance2/speedCommand ==
  r : Inport
  Compare To Constant2 : simulink/Logic and Bit Operations/Compare To Constant  relop=>  const=rp1  OutDataTypeStr=uint8  ZeroCross=off
  Gin4 : Gain  Gain=0.1  SampleTime=Tsample
  Manual Switch : ManualSwitch
  Switch : Switch  Criteria=u2 > Threshold
  Vcom : Constant  Value=Vcom  SampleTime=Tsample
  Vcom1 : Constant  Value=Vcom  SampleTime=Tsample
  Vdes : Outport
  wires:
  Manual Switch/1 -> Vdes/1
  r/1 -> Gin4/1, Compare To Constant2/1
  Gin4/1 -> Switch/3
  Switch/1 -> Manual Switch/1
  Vcom1/1 -> Manual Switch/2
  Vcom/1 -> Switch/1
  Compare To Constant2/1 -> Switch/2

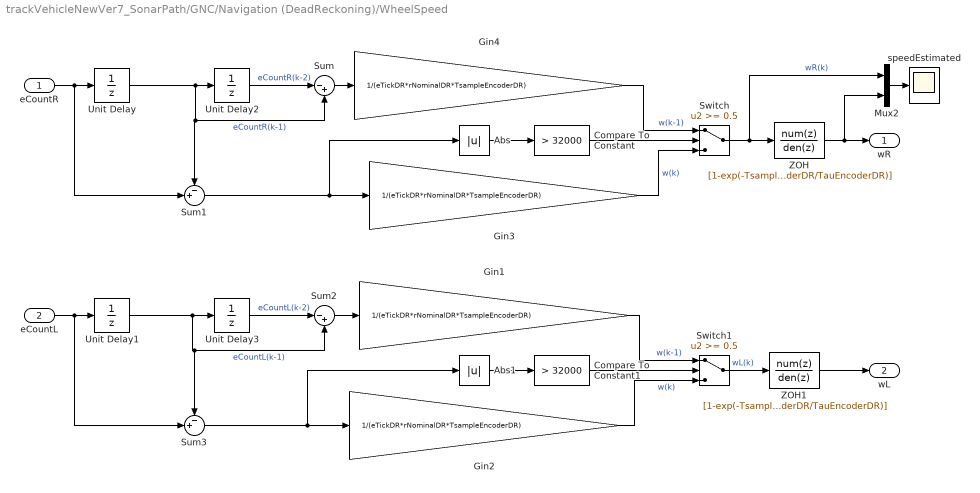
== system trackVehicleNewVer7_SonarPath/GNC/Navigation (DeadReckoning)/WheelSpeed ==
  eCountR : Inport
  eCountL : Inport  Port=2
  Abs : Abs
  Abs1 : Abs
  Compare To Constant : simulink/Logic and Bit Operations/Compare To Constant  relop=>  const=32000  OutDataTypeStr=uint8  ZeroCross=off
  Compare To Constant1 : simulink/Logic and Bit Operations/Compare To Constant  relop=>  const=32000  OutDataTypeStr=uint8  ZeroCross=off
  Gin{1..4} (4 alike) : Gain  Gain=1/(eTickDR*rNominalDR*TsampleEncoderDR)  OutDataTypeStr=double  SampleTime=TsampleEncoderDR
  Mux2 : Mux  Inputs=2
  Sum : Sum  Inputs=|-+
  Sum1 : Sum  Inputs=-+|
  Sum2 : Sum  Inputs=|-+
  Sum3 : Sum  Inputs=-+|
  Switch : Switch  Threshold=0.5
  Switch1 : Switch  Threshold=0.5
  Unit Delay{,1..3} (4 alike) : UnitDelay  SampleTime=TsampleEncoderDR
  ZOH : DiscreteTransferFcn  Numerator=[1-exp(-TsampleEncoderDR/TauEncoderDR)]  Denominator="[1  -exp(-TsampleEncoderDR/TauEncoderDR)]"  SampleTime=TsampleEncoderDR
  ZOH1 : DiscreteTransferFcn  Numerator=[1-exp(-TsampleEncoderDR/TauEncoderDR)]  Denominator="[1  -exp(-TsampleEncoderDR/TauEncoderDR)]"  SampleTime=TsampleEncoderDR
  speedEstimated : Scope
  wR : Outport
  wL : Outport  Port=2
  wires:
  eCountR/1 -> Unit Delay/1, Sum1/2
  Unit Delay/1 -> Unit Delay2/1, Sum/2, Sum1/1  "eCountR(k-1)"
  Unit Delay2/1 -> Sum/1  "eCountR(k-2)"
  Sum/1 -> Gin4/1
  Sum1/1 -> Abs/1, Gin3/1
  Gin4/1 -> Switch/1  "w(k-1)"
  Gin3/1 -> Switch/3  "w(k)"
  Abs/1 -> Compare To Constant/1
  Compare To Constant/1 -> Switch/2
  eCountL/1 -> Sum3/2, Unit Delay1/1
  Unit Delay1/1 -> Sum3/1, Sum2/2, Unit Delay3/1  "eCountL(k-1)"
  Unit Delay3/1 -> Sum2/1  "eCountL(k-2)"
  Sum2/1 -> Gin1/1
  Sum3/1 -> Abs1/1, Gin2/1
  Gin1/1 -> Switch1/1  "w(k-1)"
  Gin2/1 -> Switch1/3  "w(k)"
  Abs1/1 -> Compare To Constant1/1
  Compare To Constant1/1 -> Switch1/2
  Switch/1 -> ZOH/1, Mux2/1  "wR(k)"
  Switch1/1 -> ZOH1/1  "wL(k)"
  ZOH/1 -> wR/1, Mux2/2
  ZOH1/1 -> wL/1
  Mux2/1 -> speedEstimated/1

== system trackVehicleNewVer7_SonarPath/GNC/Guidance2/Unwrap Angle/Triggered Subsystem ==
  Trigger : TriggerPort  VariantControl=(inherit)
  Sum3 : Sum  OutDataTypeStr=int32
  Unit Delay : UnitDelay  SampleTime=-1
  countIncrement : Constant  OutDataTypeStr=int32  SampleTime=-1
  Out1 : Outport  OutDataTypeStr=int32  InitialOutput=0
  wires:
  Sum3/1 -> Unit Delay/1, Out1/1
  Unit Delay/1 -> Sum3/1
  countIncrement/1 -> Sum3/2

== system trackVehicleNewVer7_SonarPath/GNC/Guidance2/Unwrap Angle/Triggered Subsystem1 ==
  Trigger : TriggerPort  VariantControl=(inherit)
  Sum3 : Sum  Inputs=+-  OutDataTypeStr=int32
  Unit Delay : UnitDelay  SampleTime=-1
  countIncrement : Constant  OutDataTypeStr=int32  SampleTime=-1
  Out1 : Outport  OutDataTypeStr=int32  InitialOutput=0
  wires:
  countIncrement/1 -> Sum3/2
  Unit Delay/1 -> Sum3/1
  Sum3/1 -> Unit Delay/1, Out1/1

== system trackVehicleNewVer7_SonarPath/GNC/Guidance2/Waypoint Generator/Enabled Subsystem ==
  Enable : EnablePort  ZeroCross=off
  Constant : Constant
  Constant1 : Constant  Value=0
  New path flag : DataStoreWrite  DataStoreName=NewPath
  NewPath : Outport  OutputWhenDisabled=reset  InitialOutput=0
  wires:
  Constant/1 -> NewPath/1
  Constant1/1 -> New path flag/1

== matlab function trackVehicleNewVer7_SonarPath/GNC/Guidance2/MATLAB Function1 ==
  data: worldChange input; y output; newObs input; no output; pulse input
function [y,no] = fcn(worldChange, newObs,pulse)

y=0;
no=0;
persistent myTrig;

if isempty(myTrig)
    myTrig = 0;
end

if worldChange==1
    y = 1;
end
if newObs==1
    myTrig = 1;
end


if myTrig==1
    if pulse==1
        y=1;
        myTrig=0;
        no=1;
    end
end

== matlab function trackVehicleNewVer7_SonarPath/GNC/Guidance2/MATLAB Function ==
  data: trigger input; newObs output
function newObs  = fcn(trigger)
persistent trig;

if isempty(trig)
    trig = 0;
end

if trigger == 1
    if trig == 0
        newObs = 1;
        trig = 1;
    else
        newObs = 0;
    end
else 
    trig =0;
    newObs=0;
end

== matlab function trackVehicleNewVer7_SonarPath/MATLAB Function1 ==
  data: tT input; sR output; sL output
function [sR,sL] = slipFnc(tT)
%#codegen

% tT  : time
% sR  : slippage on Right Track
% sL  : slippage on Left Track

% initialization
sR=0;sL=0;

% if tT > 10 && tT < 14
%     sL=0.4;
% end
%

== matlab function trackVehicleNewVer7_SonarPath/GNC/Guidance2/Path Planner/PathPlanner ==
  data: x input; y input; heading input; goals input; OccGrid input; path output; cellsize input; gridorig input; pathlen output; newObs input; x2 output; y2 output
% Cartesian coordinate wrapper for path planner
% Start position: x, y
% Robot orientation: heading  - 0 is along the X-axis in a right-handed
% coordinate system
% goal: A list of alternative goal locations
% OccGrid: The occupancy grid - 0=Freedpace, 1=Obstacle, 2=Goal

function [path, pathlen, x2, y2] = PathPlanner(x, y, heading, goals, OccGrid, cellsize, gridorig, newObs)
path = zeros(size(OccGrid,1)*size(OccGrid,2),2);
pathlen = 0;
% Convert initial position to corresponding cell
ix = 0;
iy = 0;
[ix, iy] = pos2cell(x, y, cellsize, gridorig);
x2 = 0;
y2 = 0;

if newObs==1
    ix2=0;
    iy2=0;
    dist= 1.0;%0.6858;
    x2= x + dist*cos(heading);
    y2= y + dist*sin(heading);
    
    [ix2,iy2] = pos2cell(x2, y2, cellsize, gridorig);
     OccGrid(ix2,iy2) = 1000;
     OccGrid(ix2+1,iy2) = 1000;
     OccGrid(ix2+1,iy2-1) = 1000;
     OccGrid(ix2+1,iy2+1) = 1000;
     OccGrid(ix2,iy2+1) = 1000;
     OccGrid(ix2,iy2-1) = 1000;     
     OccGrid(ix2-1,iy2) = 1000;
     OccGrid(ix2-1,iy2+1) = 1000;     
     OccGrid(ix2-1,iy2-1) = 1000;
    % OccGrid(ix2-2,iy)=1000;
end



% Set goal states
if (size(goals, 1) > 0)
    for goalnum=1:size(goals, 1)
        [gx, gy] = pos2cell(goals(goalnum, 1), goals(goalnum, 2), cellsize, gridorig);
        OccGrid(gx, gy) = 3;
    end
    
    % Plan the path on the discrete grid
    [cellpath, cellpathlen] = planPath(ix, iy, heading, goals, OccGrid, cellsize, gridorig);

    % Set starting to beginning of the path
    path(pathlen+1,:) = [x, y]; 
    pathlen = pathlen+1; 
    if (cellpathlen > 0)   
        % Translate path into cartesian coordinates
        for step=1:cellpathlen
            [tx, ty] = cell2pos(cellpath(step,1), cellpath(step,2), cellsize, gridorig);
            path(pathlen+1,:) = [tx, ty];
            pathlen = pathlen+1;
        end
        % find nearest goal to goal bin and add it to the path as a final
        % location
        goalcell = [path(pathlen,1), path(pathlen,2)];
        mindist = Inf();
        goalindex = -1;
        for goalnum=1:size(goals, 1)
            tmpdist = sqrt((goalcell(1)-goals(goalnum,1))*(goalcell(1)-goals(goalnum,1)) + (goalcell(2)-goals(goalnum,2))*(goalcell(2)-goals(goalnum,2)));
            if (tmpdist < mindist)
                mindist = tmpdist;
                goalindex = goalnum;
            end
        end
        path(pathlen+1,:) = [goals(goalindex, 1), goals(goalindex, 2)];
        pathlen = pathlen + 1;
    end
end
path(1:pathlen,:);

end


% Path planner in grid cell coordinates
% Start grid cell: ix, iy
% Robot orientation: heading  - 0 is along the X-axis in a right-handed
% coordinate system
% OccGrid: The occupancy grid - 0=Freedpace, 1=Obstacle, 2=Goal
function [path, pathlen] = planPath(ix, iy, heading, goals, OccGrid, cellsize, gridorig)
path = zeros(size(OccGrid, 1)*size(OccGrid, 2), 2);
pathlen = 0;
gridsize = size(OccGrid);

% This is the place for the actual path planner
[gx,gy] = pos2cell(goals(1,1), goals(1,2), cellsize, gridorig);
OccGrid(gx,gy) = -3;
OccGrid(ix,iy) = -1;
OccGrid(OccGrid == 1) = 1000;
OccGrid(OccGrid == 2) = 1000;
bfsQueue = zeros(1000,2);
bfsQCount = 0;
mannOccGrid = OccGrid;

%path(1,:) = []; remove first element
%path(end+1,:) = [15,0]; reset last element as 0 0
once = 1;
n = 0;
deleter = 1;
%///////////////////// manhattan matrix
while (bfsQCount > 0 || once == 1)
   if (once == 1)
       %up
       bfsQCount = bfsQCount + 1;
       bfsQueue(bfsQCount,:) = [gx-1, gy];
       mannOccGrid(gx-1, gy) = 1;
       
       %down
       bfsQCount = bfsQCount + 1;
       bfsQueue(bfsQCount,:) = [gx+1, gy];
       mannOccGrid(gx+1, gy) = 1;

       %left
       bfsQCount = bfsQCount + 1;
       bfsQueue(bfsQCount,:) = [gx, gy-1];
       mannOccGrid(gx, gy-1) = 1;

       %right
       bfsQCount = bfsQCount + 1;
       bfsQueue(bfsQCount,:) = [gx, gy+1];
       mannOccGrid(gx, gy+1) = 1;
       once = 0;
   else
       tx = bfsQueue(deleter,1);
       ty = bfsQueue(deleter,2);
       %ismember([2,2],a,'rows')
       if mannOccGrid(tx, ty) == -1
           break;
       end
       %up
       if ((tx - 1) > 0)
           if mannOccGrid(tx-1, ty) ~= 0
               
           else
               bfsQCount = bfsQCount + 1;
               bfsQueue(deleter + bfsQCount - 1,:) = [tx-1, ty];
               mannOccGrid(tx-1, ty) = mannOccGrid(tx,ty) + 1;
           end
       end
       %down
       if ((tx + 1) <= 30)
           if mannOccGrid(tx+1, ty) ~= 0
               
           else
               bfsQCount = bfsQCount + 1;
               bfsQueue(deleter + bfsQCount - 1,:) = [tx+1, ty];
               mannOccGrid(tx+1, ty) = mannOccGrid(tx,ty) + 1;
           end
       end
       %left
       if ((ty - 1) > 0)
           if mannOccGrid(tx, ty-1) ~= 0
               
           else
               bfsQCount = bfsQCount + 1;
               bfsQueue(deleter + bfsQCount - 1,:) = [tx, ty-1];
               mannOccGrid(tx, ty-1) = mannOccGrid(tx,ty) + 1;
           end
       end
       %right
       if ((ty + 1) <= 30)
           if mannOccGrid(tx, ty+1) ~= 0
               
           else
               bfsQCount = bfsQCount + 1;
               bfsQueue(deleter + bfsQCount - 1,:) = [tx, ty+1];
               mannOccGrid(tx, ty+1) = mannOccGrid(tx,ty) + 1;
           end
       end
       %bfsQueue(1,:) = [];
       %bfsQueue(end+1,:) = [0,0];
       deleter = deleter + 1;
       bfsQCount = bfsQCount - 1;
   end
   n = n+1;
end
%///////////////////// shortest path
flpOccGrid = mannOccGrid;%flip(mannOccGrid);
ox = ix;
oy = iy;
n = 0;
m=0;
pathM = zeros(100,2);
while (flpOccGrid(ox,oy) ~= -3)
    v1 = 500; %up
    v2 = 500; %down
    v3 = 500; %left
    v4 = 500; %right
    if flpOccGrid(ox, oy) == -3
        break;
    end
   if ((ox - 1) > 0)
       if and(flpOccGrid(ox-1, oy) ~= 1000 , flpOccGrid(ox-1, oy) ~= -1)
           v1 = flpOccGrid(ox-1, oy);
       end
   end
   if ((ox + 1) <= 30)
       if and(flpOccGrid(ox+1, oy) ~= 1000 , flpOccGrid(ox+1, oy) ~= -1)
           v2 = flpOccGrid(ox+1, oy);
       end
   end
   if ((oy - 1) > 0)
       if and(flpOccGrid(ox, oy-1) ~= 1000 , flpOccGrid(ox, oy-1) ~= -1)
           v3 = flpOccGrid(ox, oy-1);
       end
   end
   if ((oy + 1) <= 30)
       if and(flpOccGrid(ox, oy+1) ~= 1000 , flpOccGrid(ox, oy+1) ~= -1)
           v4 = flpOccGrid(ox, oy+1);
       end
   end
    tmp = [v1,v2,v3,v4];
    tmp1 = find(tmp == min(tmp));
    val = tmp1(1,1);
    switch val
        case 1
            ox = ox - 1;
            oy = oy;
            m = n+1;
            pathM(m,1) = ox;
            pathM(m,2) = oy;
        case 2
            ox = ox + 1;
            oy = oy;
            m = n+1;
            pathM(m,:) = [ox,oy];
        case 3
            ox = ox;
            oy = oy - 1;
            m = n+1;
            pathM(m,:) = [ox,oy];
        case 4
            ox = ox;
            oy = oy + 1;
            m = n+1;
            pathM(m,:) = [ox,oy];
    end
    n = n+1;
end
path = pathM;
pathlen = n;
end



% Converts cartesian position into grid cell index
function [ix, iy] = pos2cell(x, y, cellsize, gridorig)
ix = max(floor((x - gridorig(1))/cellsize(1))+1, 1);
iy = max(floor((y - gridorig(2))/cellsize(2))+1, 1);
end

%Converts grid cell index into cartesian position
function [x, y] = cell2pos(ix, iy, cellsize, gridorig)
x = (ix-0.5) * cellsize(1) + gridorig(1);
y = (iy-0.5) * cellsize(2) + gridorig(2);
end

== matlab function trackVehicleNewVer7_SonarPath/GNC/Guidance2/Waypoint Generator/Waypoint Sequencer ==
  data: x input; y input; path input; xway output; yway output; pathlen input; pathidx input; wayidx output; newpath input; stop output; maxwaydist input; maxgoaldist input
function [xway, yway, wayidx, stop] = NextWaypoint(x, y, path, pathlen, pathidx, newpath, maxwaydist, maxgoaldist)
xway = 0.0;
yway = 0.0;
wayidx = pathidx;
stop = 0;

if (pathlen > 0)
    if (newpath)
        wayidx = 1;
    end
    currdist = sqrt((path(wayidx, 1)-x)*(path(wayidx, 1)-x) + (path(wayidx, 2)-y)*(path(wayidx, 2)-y));
    if ( currdist < maxwaydist)
        if (wayidx == pathlen)
            if (currdist < maxgoaldist) 
                stop = 1;
            end
        else
            wayidx = wayidx + 1; 
        end
    end
    xway = path(wayidx, 1);
    yway = path(wayidx, 2);        
else
    xway = x;
    yway = y;
    stop = 0;
end
end

== matlab function trackVehicleNewVer7_SonarPath/Tank/MATLAB Function2 ==
  data: u input; x_dot output; b parameter; rr parameter; rl parameter
function x_dot = fcn(u,b,rr,rl)
%#codegen

wr = u(1);
wl = u(2);
theta = u(3);
sr = u(4);
sl = u(5);
x_dot = [((1-sl)*rl*wl + (1-sr)*rr*wr)*cos(theta)/2;
         ((1-sl)*rl*wl + (1-sr)*rr*wr)*sin(theta)/2;
         ((1-sl)*rl*wl - (1-sr)*rr*wr)/b];

== matlab function trackVehicleNewVer7_SonarPath/Tank/MATLAB Function3 ==
  data: obstacles input; rObst output; xUGV input; yUGV input; aUGV input; sonarInfo parameter
function rObst = sonarRange(obstacles,xUGV,yUGV,aUGV,sonarInfo)
%#codegen

% obstacles : Matrix 3Xn, n is the number of obstacles
% obstacles(1,:): x-position of obstacles [m]
% obstacles(2,:): y-position of obstacles [m]
% obstacles(3,:): radious of obstacles [m]

% xUGV:  x-position of UGV [m]
% yUGV:  y-position of UGV [m]
% aUGV: orientation of UGV [rad]


% sonarInfo.as : width of the sensor coveragle [m]
% sonarInfo.bs : length of the sensor coveragle [m]
% sonarInfo.hs : position of the sensor coveragle [m] (offset longitudinally from the origin of the body-frame)

% rObst: range of the obstacle measured by the sonar sensor [cm] !!!! note
% the unit.  unit is cm because that is what the actual sensor readings are

rObst = 7.67; % default sensor output when there is no detection

RBI = [cos(aUGV) sin(aUGV);-sin(aUGV) cos(aUGV)];


temp =size(obstacles);
noOfObst = temp(2);
for indexObst = 1:noOfObst
    
    rhoXYobst = RBI*(obstacles(1:2,indexObst)-[xUGV;yUGV]);
    
    obstXup    = rhoXYobst(1)+obstacles(3,indexObst);
    obstXdown  = rhoXYobst(1)-obstacles(3,indexObst);
    obstYright = rhoXYobst(2)+obstacles(3,indexObst);
    obstYleft  = rhoXYobst(2)-obstacles(3,indexObst);
    
    sonarXup    =  sonarInfo.hs + sonarInfo.bs;
    sonarXdown  =  sonarInfo.hs;
    sonarYright =  sonarInfo.as/2;
    sonarYleft  = -sonarInfo.as/2;
    
    flgOLx = overlapCheck([obstXdown obstXup],[sonarXdown sonarXup]);
    flgOLy = overlapCheck([obstYleft obstYright],[sonarYleft sonarYright]);
    
    if flgOLx && flgOLy
        temp2 = max(0,rhoXYobst(1) - obstacles(3,indexObst) - sonarInfo.hs);
        rObst = min(temp2,rObst);
    end
end
rObst = 100*rObst;


function [flgOL]=overlapCheck(aa,bb)
%#codegen
% checks if there is overlap between two intervals (aa(1),aa(2)) and (bb(1),bb(3))
% flgOL = 0 => no overlap, flgOL = 1 => overlap
% Dogan, 20150403

flgOL = 0;
if aa(1) <= bb(1)
    left = aa;
    right = bb;
else
    left = bb;
    right = aa;
end

if left(2) >= right(1)
    flgOL = 1;
end
